simulink model "microgrid_y22s_step2"  (R2021b)
settings: Solver=ode45  StartTime=0.0  StopTime=10  FixedStep=0.5  MaxStep=1e-3  RelTol=1e-3
values from neighbouring files (symbols this model uses):
  A = pi*bladeLength^2    (= 5026.54824574)    [firstinitialization.m]
  bladeLength = 40    [firstinitialization.m]
  J = 100e3    (= 100000)    [firstinitialization.m]
  Kfric = 27    [firstinitialization.m]
  rho = 1.2    [firstinitialization.m]
settings Model: Creator=tedbrekken  LastModifiedBy=tedbrekken
settings SolverCC: AlgebraicLoopSolver=TrustRegion
settings DataIOCC: ReturnWorkspaceOutputs=off
settings DebuggingCC: SFMachineParentedDataDiag=warning

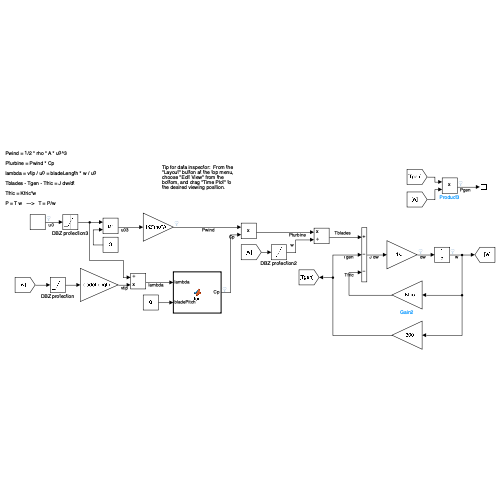
[thumbnail: Simulink's stored preview of the top-level diagram]
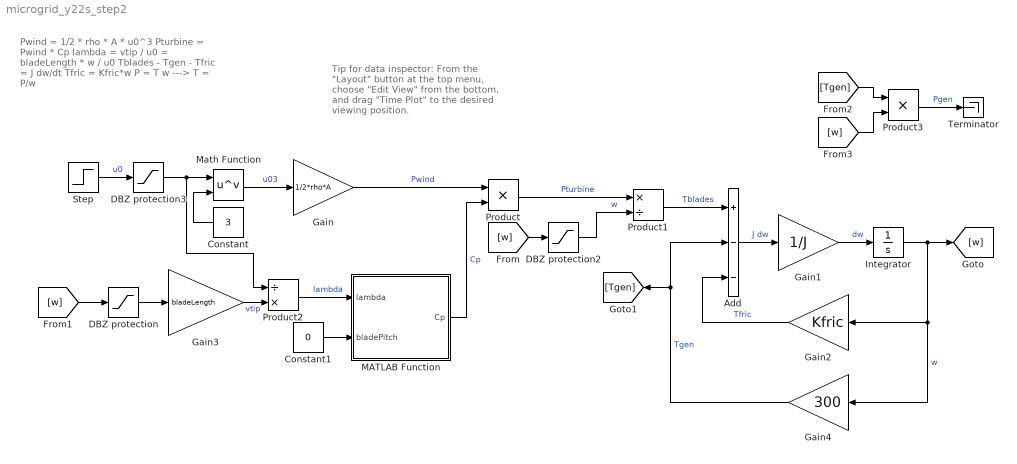
== system microgrid_y22s_step2 ==
  note: Tip for data inspector: From the "Layout" button at the top menu, choose "Edit View" from the bottom, and drag "Time Plot" to the desired viewing position.
  note: Pwind = 1/2 * rho * A * u0^3
      |
      | Pturbine = Pwind * Cp
      |
      | lambda = vtip / u0 = bladeLength * w / u0
      |
      | Tblades - Tgen - Tfric = J dw/dt
      |
      | Tfric = Kfric*w
      |
      | P = T w   --->   T = P/w
  Add : Sum  Inputs=+--
  Constant : Constant  Value=3
  Constant1 : Constant  Value=0
  DBZ protection : Saturate  UpperLimit=inf  LowerLimit=0.001
  DBZ protection2 : Saturate  UpperLimit=inf  LowerLimit=0.001
  DBZ protection3 : Saturate  UpperLimit=inf  LowerLimit=0.001
  Gain : Gain  Gain=1/2*rho*A
  Gain1 : Gain  Gain=1/J
  Gain2 : Gain  Gain=Kfric
  Gain3 : Gain  Gain=bladeLength
  Gain4 : Gain  Gain=300
  Integrator : Integrator
  MATLAB Function : MATLAB Function  TreatAsAtomicUnit=on
  Math Function : Math  Operator=pow  SaturateOnIntegerOverflow=on
  Product : Product
  Product1 : Product  Inputs=*/
  Product2 : Product  Inputs=/*
  Product3 : Product
  Step : Step  Time=5  Before=5  After=7  SampleTime=0
  Terminator : Terminator
  wires:
  Math Function/1 -> Gain/1  "u03"
  Gain/1 -> Product/1  "Pwind"
  Step/1 -> DBZ protection3/1  "u0"
  Constant/1 -> Math Function/2
  MATLAB Function/1(Cp) -> Product/2  "Cp"
  Product/1 -> Product1/1  "Pturbine"
  Product1/1 -> Add/1  "Tblades"
  Integrator/1 -> Gain4/1, Gain2/1, [w]  "w"
  Gain4/1 -> [Tgen], Add/2  "Tgen"
  Gain2/1 -> Add/3  "Tfric"
  Add/1 -> Gain1/1  "J dw"
  Gain1/1 -> Integrator/1  "dw"
  DBZ protection2/1 -> Product1/2  "w"
  [w] -> DBZ protection/1
  Gain3/1 -> Product2/2  "vtip"
  Product2/1 -> MATLAB Function/1(lambda)  "lambda"
  Constant1/1 -> MATLAB Function/2(bladePitch)
  [w] -> DBZ protection2/1
  DBZ protection/1 -> Gain3/1
  DBZ protection3/1 -> Product2/1, Math Function/1
  [Tgen] -> Product3/1
  [w] -> Product3/2
  Product3/1 -> Terminator/1  "Pgen"

== matlab function microgrid_y22s_step2/MATLAB Function ==
  data: lambda input; Cp output; bladePitch input
function Cp = fcn(lambda,bladePitch)

% https://www.mathworks.com/help/physmod/sps/powersys/ref/windturbine.html

c = [...
    0.5176 ...
    116 ...
    0.4 ...
    5 ...
    21 ...
    0.0068];

lambdaai = 1/( 1/(lambda+0.08*bladePitch) - 0.035/(bladePitch^3+1) );

Cp = c(1)*(c(2)/lambdaai-c(3)*bladePitch-c(4))*exp(-c(5)/lambdaai) + c(6)*lambda;
